simulink model "paper1_cs"  (R2021b)
settings: Solver=ode4  StartTime=0.0  StopTime=120  FixedStep=1/20  RelTol=1e-3
PreLoadFcn:
  | mbxruntime.callbacks.PreLoadFcn(bdroot);
PostLoadFcn:
  | mbxruntime.callbacks.PostLoadFcn(bdroot);
InitFcn:
  | mbxruntime.callbacks.InitFcn(bdroot);
StartFcn:
  | mbxruntime.callbacks.StartFcn(bdroot);
StopFcn:
  | mbxruntime.callbacks.StopFcn(bdroot);
model workspace (MAT data in the model file):
  mbox_table : object (value not decoded)
  model_closed = 0
  sim_status = 0
undefined symbols (not defined in the file): DiscIntNeverNeededParam
libraries: PreScanSimulinkLibrary x12, Solver_SF x6, simulink x1
(part 3 of 3)

== system paper1_cs/Audi_A8_Sedan_5/SELF_Demux ==
  SELF : Inport  OutDataTypeStr=Bus: PRESCAN_SELFSENSORDATA
  Bus Selector : BusSelector  OutputSignals=PositionX,PositionY,PositionZ,OrientationRoll,OrientationPitch,OrientationYaw,Velocity,Yaw_rate,Lat,Long,Alt
  Demux2 : Demux  Outputs=3
  Gain : Gain  Gain=180/pi
  Gain1 : Gain  Gain=180/pi
  Vector Concatenate1 : Concatenate  NumInputs=3
  compas converter : Subsystem
  x [m] : Outport
  y [m] : Outport  Port=2
  z [m] : Outport  Port=3
  rotx [deg] : Outport  Port=4
  roty [deg] : Outport  Port=5
  rotz [deg] : Outport  Port=6
  GPS lat [deg] : Outport  Port=7
  GPS long [deg] : Outport  Port=8
  GPS alt [m] : Outport  Port=9
  velocity [m/s] : Outport  Port=10
  heading [deg] : Outport  Port=11
  yaw rate [deg/s] : Outport  Port=12
  wires:
  Bus Selector/11 -> GPS alt [m]/1  "<Alt>"
  Bus Selector/10 -> GPS long [deg]/1  "<Long>"
  Bus Selector/9 -> GPS lat [deg]/1  "<Lat>"
  Bus Selector/8 -> Gain1/1  "<Yaw_rate>"
  Bus Selector/7 -> velocity [m/s]/1  "<Velocity>"
  Bus Selector/6 -> compas converter/1(rotz [rad]), Vector Concatenate1/3  "<OrientationYaw>"
  Bus Selector/5 -> Vector Concatenate1/2  "<OrientationPitch>"
  Bus Selector/4 -> Vector Concatenate1/1  "<OrientationRoll>"
  Vector Concatenate1/1 -> Gain/1
  Bus Selector/3 -> z [m]/1  "<PositionZ>"
  Bus Selector/2 -> y [m]/1  "<PositionY>"
  Bus Selector/1 -> x [m]/1  "<PositionX>"
  SELF/1 -> Bus Selector/1
  Gain/1 -> Demux2/1
  Demux2/1 -> rotx [deg]/1
  Demux2/2 -> roty [deg]/1
  Demux2/3 -> rotz [deg]/1
  compas converter/1(heading [deg]) -> heading [deg]/1
  Gain1/1 -> yaw rate [deg/s]/1

== system paper1_cs/Audi_A8_Sedan_5/STATE_Audi_A8_Sedan_5 ==
  State : Inport  SampleTime=TimeStep
  Bus Creator : BusCreator  Inputs=15  OutDataTypeStr=Bus: PRESCAN_STATEACTUATORDATA  NonVirtualBus=on
  Demux : Demux  Outputs=15
  iniBODYAngles wrtVEH [rad] : Constant  Value=[Roll0 Pitch0 0]  SampleTime=TimeStep
  iniVEHAngles wrtGLOB [rad] : Constant  Value=[0 0 Yaw0]  SampleTime=TimeStep
  iniVEHposition wrtGLOB [m] : Constant  Value=[x0 y0 z0]  SampleTime=TimeStep
  state2FullState : PreScanSimulinkLibrary/state2FullState  SystemSampleTime=-1  VariantActivationTime=update diagram  Latency=0  AutoFrameSizeCalculation=off
  StateBus : Outport  OutDataTypeStr=Bus: PRESCAN_STATEACTUATORDATA
  wires:
  Bus Creator/1 -> StateBus/1
  State/1 -> state2FullState/1
  state2FullState/1 -> Demux/1
  iniVEHposition wrtGLOB [m]/1 -> state2FullState/2
  iniBODYAngles wrtVEH [rad]/1 -> state2FullState/3
  iniVEHAngles wrtGLOB [rad]/1 -> state2FullState/4
  Demux/1 -> Bus Creator/1  "PositionX"
  Demux/2 -> Bus Creator/2  "PositionY"
  Demux/3 -> Bus Creator/3  "PositionZ"
  Demux/4 -> Bus Creator/4  "VelocityX"
  Demux/5 -> Bus Creator/5  "VelocityY"
  Demux/6 -> Bus Creator/6  "VelocityZ"
  Demux/7 -> Bus Creator/7  "AccelerationX"
  Demux/8 -> Bus Creator/8  "AccelerationY"
  Demux/9 -> Bus Creator/9  "AccelerationZ"
  Demux/10 -> Bus Creator/10  "OrientationRoll"
  Demux/11 -> Bus Creator/11  "OrientationPitch"
  Demux/12 -> Bus Creator/12  "OrientationYaw"
  Demux/13 -> Bus Creator/13  "AngularVelocityRoll"
  Demux/14 -> Bus Creator/14  "AngularVelocityPitch"
  Demux/15 -> Bus Creator/15  "AngularVelocityYaw"

== system paper1_cs/Audi_A8_Sedan_6/Dynamics_UserSpecified ==
  note: For state mode 'Dynamic' positions
      | are not taken into account, as they
      | are computed by integrating velocity.
      | Click annotation for Help.
  CarSim S-Function : Solver_SF/CarSim S-Function  Priority=1  Commented=on  SIMFILE=simfile.sim  Run_RTs=off  vs_state_ind=Run  StopMode_ind=Vehicle Model
  Ground1 : Ground
  MuxState : Subsystem  Tag=mux/State  mask(Empty Dynamics State Block){positioningmode=on, TimeStep=1/20}
      mask prompts: positioningmode "Positioning Mode"; TimeStep "Auto Assigned: Time Step [s]"
      mask help:
      | Build the state of an actor based on user input.
      | The user can either use positioning mode or dynamics mode.
      | - When using positioning mode the position and orientation of the actor are set directly based on the input. Expected input is relative to the initial position and orientation of the actor. It's also possible to specify the velocity of the actor, though this input isn't used, only passed on.
      | - When using dynamics mode the position input is ignored. Expected input is velocity and orientation. The velocity is relative the current orientation of the actor, while orientation is relative to its initial orientation. The position of the actor is calculated based on the velocity and orientation given.
      settings: DeleteFcn=PreScanBlockDeleteFcn;
  State : Outport
  wires:
  [v6] -> MuxState/4(dx [m/s])
  [x6] -> MuxState/1(x [m])
  MuxState/1(state) -> State/1
  Ground1/1 -> MuxState/2(y [m]), MuxState/3(z [m]), MuxState/5(dy [m/s]), MuxState/6(dz [m/s]), MuxState/7(R [rad]), MuxState/8(P [rad]), MuxState/9(Y [rad])

== system paper1_cs/Audi_A8_Sedan_6/SELF_Demux ==
  SELF : Inport  OutDataTypeStr=Bus: PRESCAN_SELFSENSORDATA
  Bus Selector : BusSelector  OutputSignals=PositionX,PositionY,PositionZ,OrientationRoll,OrientationPitch,OrientationYaw,Velocity,Yaw_rate,Lat,Long,Alt
  Demux2 : Demux  Outputs=3
  Gain : Gain  Gain=180/pi
  Gain1 : Gain  Gain=180/pi
  Vector Concatenate1 : Concatenate  NumInputs=3
  compas converter : Subsystem
  x [m] : Outport
  y [m] : Outport  Port=2
  z [m] : Outport  Port=3
  rotx [deg] : Outport  Port=4
  roty [deg] : Outport  Port=5
  rotz [deg] : Outport  Port=6
  GPS lat [deg] : Outport  Port=7
  GPS long [deg] : Outport  Port=8
  GPS alt [m] : Outport  Port=9
  velocity [m/s] : Outport  Port=10
  heading [deg] : Outport  Port=11
  yaw rate [deg/s] : Outport  Port=12
  wires:
  Bus Selector/11 -> GPS alt [m]/1  "<Alt>"
  Bus Selector/10 -> GPS long [deg]/1  "<Long>"
  Bus Selector/9 -> GPS lat [deg]/1  "<Lat>"
  Bus Selector/8 -> Gain1/1  "<Yaw_rate>"
  Bus Selector/7 -> velocity [m/s]/1  "<Velocity>"
  Bus Selector/6 -> compas converter/1(rotz [rad]), Vector Concatenate1/3  "<OrientationYaw>"
  Bus Selector/5 -> Vector Concatenate1/2  "<OrientationPitch>"
  Bus Selector/4 -> Vector Concatenate1/1  "<OrientationRoll>"
  Vector Concatenate1/1 -> Gain/1
  Bus Selector/3 -> z [m]/1  "<PositionZ>"
  Bus Selector/2 -> y [m]/1  "<PositionY>"
  Bus Selector/1 -> x [m]/1  "<PositionX>"
  SELF/1 -> Bus Selector/1
  Gain/1 -> Demux2/1
  Demux2/1 -> rotx [deg]/1
  Demux2/2 -> roty [deg]/1
  Demux2/3 -> rotz [deg]/1
  compas converter/1(heading [deg]) -> heading [deg]/1
  Gain1/1 -> yaw rate [deg/s]/1

== system paper1_cs/Audi_A8_Sedan_6/STATE_Audi_A8_Sedan_6 ==
  State : Inport  SampleTime=TimeStep
  Bus Creator : BusCreator  Inputs=15  OutDataTypeStr=Bus: PRESCAN_STATEACTUATORDATA  NonVirtualBus=on
  Demux : Demux  Outputs=15
  iniBODYAngles wrtVEH [rad] : Constant  Value=[Roll0 Pitch0 0]  SampleTime=TimeStep
  iniVEHAngles wrtGLOB [rad] : Constant  Value=[0 0 Yaw0]  SampleTime=TimeStep
  iniVEHposition wrtGLOB [m] : Constant  Value=[x0 y0 z0]  SampleTime=TimeStep
  state2FullState : PreScanSimulinkLibrary/state2FullState  SystemSampleTime=-1  VariantActivationTime=update diagram  Latency=0  AutoFrameSizeCalculation=off
  StateBus : Outport  OutDataTypeStr=Bus: PRESCAN_STATEACTUATORDATA
  wires:
  Bus Creator/1 -> StateBus/1
  State/1 -> state2FullState/1
  state2FullState/1 -> Demux/1
  iniVEHposition wrtGLOB [m]/1 -> state2FullState/2
  iniBODYAngles wrtVEH [rad]/1 -> state2FullState/3
  iniVEHAngles wrtGLOB [rad]/1 -> state2FullState/4
  Demux/1 -> Bus Creator/1  "PositionX"
  Demux/2 -> Bus Creator/2  "PositionY"
  Demux/3 -> Bus Creator/3  "PositionZ"
  Demux/4 -> Bus Creator/4  "VelocityX"
  Demux/5 -> Bus Creator/5  "VelocityY"
  Demux/6 -> Bus Creator/6  "VelocityZ"
  Demux/7 -> Bus Creator/7  "AccelerationX"
  Demux/8 -> Bus Creator/8  "AccelerationY"
  Demux/9 -> Bus Creator/9  "AccelerationZ"
  Demux/10 -> Bus Creator/10  "OrientationRoll"
  Demux/11 -> Bus Creator/11  "OrientationPitch"
  Demux/12 -> Bus Creator/12  "OrientationYaw"
  Demux/13 -> Bus Creator/13  "AngularVelocityRoll"
  Demux/14 -> Bus Creator/14  "AngularVelocityPitch"
  Demux/15 -> Bus Creator/15  "AngularVelocityYaw"

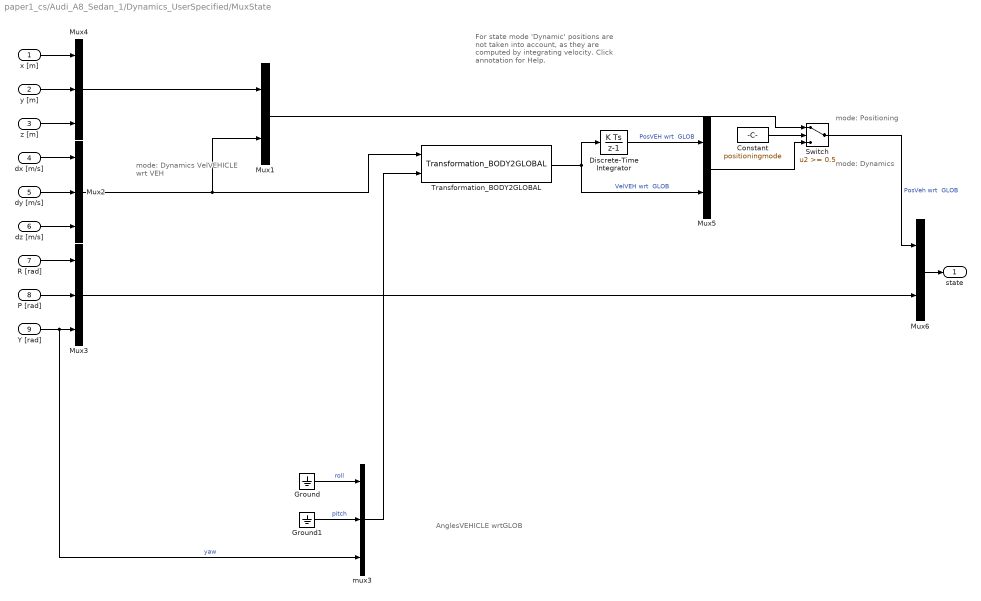
== system paper1_cs/Audi_A8_Sedan_1/Dynamics_UserSpecified/MuxState ==
  note: mode: Dynamics
  note: mode: Positioning
  note: mode: Dynamics
      | VelVEHICLE
      | wrt VEH
  note: AnglesVEHICLE
      | wrtGLOB
  note: For state mode 'Dynamic' positions
      | are not taken into account, as they
      | are computed by integrating velocity.
      | Click annotation for Help.
  x [m] : Inport  SampleTime=TimeStep
  y [m] : Inport  Port=2  SampleTime=TimeStep
  z [m] : Inport  Port=3  SampleTime=TimeStep
  dx [m/s] : Inport  Port=4  SampleTime=TimeStep
  dy [m/s] : Inport  Port=5  SampleTime=TimeStep
  dz [m/s] : Inport  Port=6  SampleTime=TimeStep
  R [rad] : Inport  Port=7  SampleTime=TimeStep
  P [rad] : Inport  Port=8  SampleTime=TimeStep
  Y [rad] : Inport  Port=9  SampleTime=TimeStep
  Constant : Constant  DisableCoverage=on  Value=positioningmode
  Discrete-Time Integrator : DiscreteIntegrator  SampleTime=TimeStep  ICPrevOutput=DiscIntNeverNeededParam  ICPrevScaledInput=DiscIntNeverNeededParam
  Ground : Ground
  Ground1 : Ground
  Mux1 : Mux  Inputs=[3 3]
  Mux2 : Mux  Inputs=3
  Mux3 : Mux  Inputs=3
  Mux4 : Mux  Inputs=3
  Mux5 : Mux  Inputs=[3 3]
  Mux6 : Mux  Inputs=[6 3]
  Switch : Switch  Threshold=0.5
  Transformation_BODY2GLOBAL : PreScanSimulinkLibrary/Simple_Vehicle_Dynamics/Chassis/MuxDynState/Transformation_BODY2GLOBAL  SystemSampleTime=-1  VariantActivationTime=update diagram  Latency=0  AutoFrameSizeCalculation=off
  mux3 : Mux  Inputs=3
  state : Outport
  wires:
  Constant/1 -> Switch/2
  Mux6/1 -> state/1
  Mux4/1 -> Mux1/1
  Mux5/1 -> Switch/3
  Mux1/1 -> Switch/1
  Switch/1 -> Mux6/1  "PosVeh wrt  GLOB"
  P [rad]/1 -> Mux3/2
  R [rad]/1 -> Mux3/1
  dz [m/s]/1 -> Mux2/3
  dy [m/s]/1 -> Mux2/2
  dx [m/s]/1 -> Mux2/1
  z [m]/1 -> Mux4/3
  y [m]/1 -> Mux4/2
  x [m]/1 -> Mux4/1
  Ground1/1 -> mux3/2  "pitch"
  Y [rad]/1 -> mux3/3, Mux3/3  "yaw"
  Mux3/1 -> Mux6/2
  Transformation_BODY2GLOBAL/1 -> Discrete-Time Integrator/1, Mux5/2  "VelVEH wrt  GLOB"
  mux3/1 -> Transformation_BODY2GLOBAL/2
  Ground/1 -> mux3/1  "roll"
  Mux2/1 -> Mux1/2, Transformation_BODY2GLOBAL/1
  Discrete-Time Integrator/1 -> Mux5/1  "PosVEH wrt  GLOB"

== system paper1_cs/Audi_A8_Sedan_1/SELF_Demux/compas converter ==
  rotz [rad] : Inport
  cart2compas : Subsystem
  rad2deg : Gain  Gain=180/pi
  heading [deg] : Outport
  wires:
  rad2deg/1 -> cart2compas/1(Angle [deg])
  rotz [rad]/1 -> rad2deg/1
  cart2compas/1(heading [deg]) -> heading [deg]/1

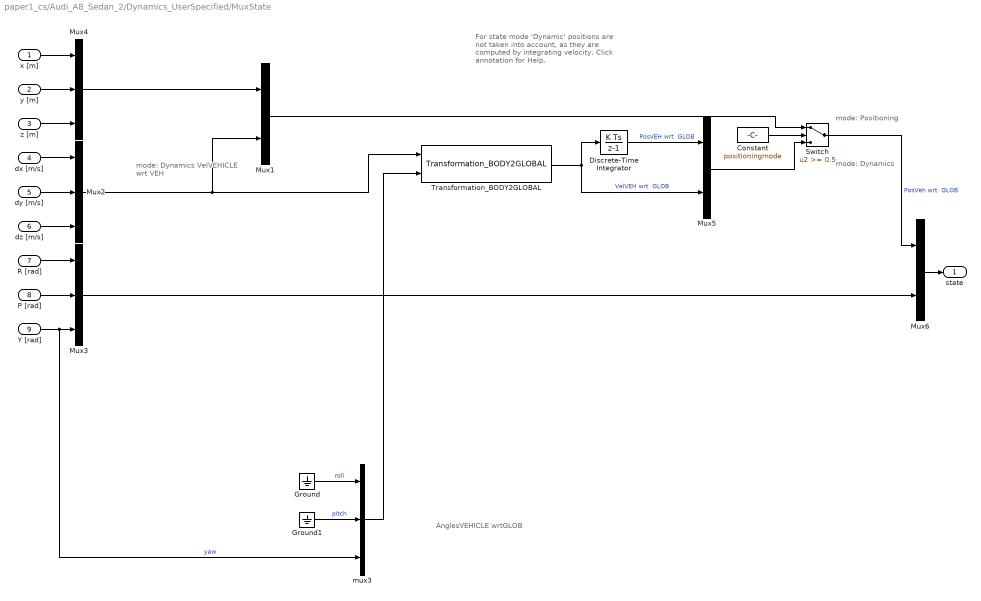
== system paper1_cs/Audi_A8_Sedan_2/Dynamics_UserSpecified/MuxState ==
  note: mode: Dynamics
  note: mode: Positioning
  note: mode: Dynamics
      | VelVEHICLE
      | wrt VEH
  note: AnglesVEHICLE
      | wrtGLOB
  note: For state mode 'Dynamic' positions
      | are not taken into account, as they
      | are computed by integrating velocity.
      | Click annotation for Help.
  x [m] : Inport  SampleTime=TimeStep
  y [m] : Inport  Port=2  SampleTime=TimeStep
  z [m] : Inport  Port=3  SampleTime=TimeStep
  dx [m/s] : Inport  Port=4  SampleTime=TimeStep
  dy [m/s] : Inport  Port=5  SampleTime=TimeStep
  dz [m/s] : Inport  Port=6  SampleTime=TimeStep
  R [rad] : Inport  Port=7  SampleTime=TimeStep
  P [rad] : Inport  Port=8  SampleTime=TimeStep
  Y [rad] : Inport  Port=9  SampleTime=TimeStep
  Constant : Constant  DisableCoverage=on  Value=positioningmode
  Discrete-Time Integrator : DiscreteIntegrator  SampleTime=TimeStep  ICPrevOutput=DiscIntNeverNeededParam  ICPrevScaledInput=DiscIntNeverNeededParam
  Ground : Ground
  Ground1 : Ground
  Mux1 : Mux  Inputs=[3 3]
  Mux2 : Mux  Inputs=3
  Mux3 : Mux  Inputs=3
  Mux4 : Mux  Inputs=3
  Mux5 : Mux  Inputs=[3 3]
  Mux6 : Mux  Inputs=[6 3]
  Switch : Switch  Threshold=0.5
  Transformation_BODY2GLOBAL : PreScanSimulinkLibrary/Simple_Vehicle_Dynamics/Chassis/MuxDynState/Transformation_BODY2GLOBAL  SystemSampleTime=-1  VariantActivationTime=update diagram  Latency=0  AutoFrameSizeCalculation=off
  mux3 : Mux  Inputs=3
  state : Outport
  wires:
  Constant/1 -> Switch/2
  Mux6/1 -> state/1
  Mux4/1 -> Mux1/1
  Mux5/1 -> Switch/3
  Mux1/1 -> Switch/1
  Switch/1 -> Mux6/1  "PosVeh wrt  GLOB"
  P [rad]/1 -> Mux3/2
  R [rad]/1 -> Mux3/1
  dz [m/s]/1 -> Mux2/3
  dy [m/s]/1 -> Mux2/2
  dx [m/s]/1 -> Mux2/1
  z [m]/1 -> Mux4/3
  y [m]/1 -> Mux4/2
  x [m]/1 -> Mux4/1
  Ground1/1 -> mux3/2  "pitch"
  Y [rad]/1 -> mux3/3, Mux3/3  "yaw"
  Mux3/1 -> Mux6/2
  Transformation_BODY2GLOBAL/1 -> Discrete-Time Integrator/1, Mux5/2  "VelVEH wrt  GLOB"
  mux3/1 -> Transformation_BODY2GLOBAL/2
  Ground/1 -> mux3/1  "roll"
  Mux2/1 -> Mux1/2, Transformation_BODY2GLOBAL/1
  Discrete-Time Integrator/1 -> Mux5/1  "PosVEH wrt  GLOB"

== system paper1_cs/Audi_A8_Sedan_2/SELF_Demux/compas converter ==
  rotz [rad] : Inport
  cart2compas : Subsystem
  rad2deg : Gain  Gain=180/pi
  heading [deg] : Outport
  wires:
  rad2deg/1 -> cart2compas/1(Angle [deg])
  rotz [rad]/1 -> rad2deg/1
  cart2compas/1(heading [deg]) -> heading [deg]/1

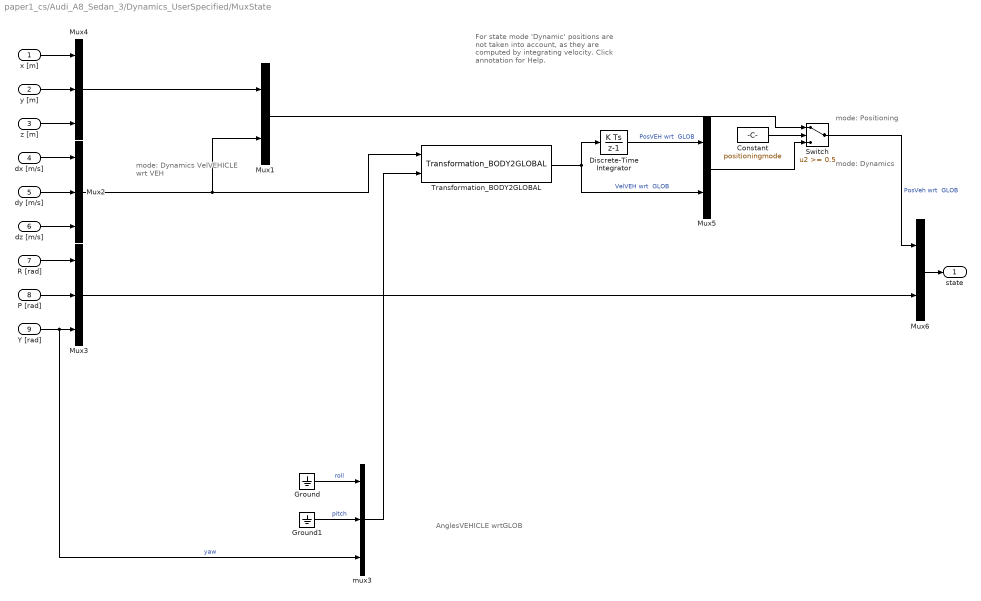
== system paper1_cs/Audi_A8_Sedan_3/Dynamics_UserSpecified/MuxState ==
  note: mode: Dynamics
  note: mode: Positioning
  note: mode: Dynamics
      | VelVEHICLE
      | wrt VEH
  note: AnglesVEHICLE
      | wrtGLOB
  note: For state mode 'Dynamic' positions
      | are not taken into account, as they
      | are computed by integrating velocity.
      | Click annotation for Help.
  x [m] : Inport  SampleTime=TimeStep
  y [m] : Inport  Port=2  SampleTime=TimeStep
  z [m] : Inport  Port=3  SampleTime=TimeStep
  dx [m/s] : Inport  Port=4  SampleTime=TimeStep
  dy [m/s] : Inport  Port=5  SampleTime=TimeStep
  dz [m/s] : Inport  Port=6  SampleTime=TimeStep
  R [rad] : Inport  Port=7  SampleTime=TimeStep
  P [rad] : Inport  Port=8  SampleTime=TimeStep
  Y [rad] : Inport  Port=9  SampleTime=TimeStep
  Constant : Constant  DisableCoverage=on  Value=positioningmode
  Discrete-Time Integrator : DiscreteIntegrator  SampleTime=TimeStep  ICPrevOutput=DiscIntNeverNeededParam  ICPrevScaledInput=DiscIntNeverNeededParam
  Ground : Ground
  Ground1 : Ground
  Mux1 : Mux  Inputs=[3 3]
  Mux2 : Mux  Inputs=3
  Mux3 : Mux  Inputs=3
  Mux4 : Mux  Inputs=3
  Mux5 : Mux  Inputs=[3 3]
  Mux6 : Mux  Inputs=[6 3]
  Switch : Switch  Threshold=0.5
  Transformation_BODY2GLOBAL : PreScanSimulinkLibrary/Simple_Vehicle_Dynamics/Chassis/MuxDynState/Transformation_BODY2GLOBAL  SystemSampleTime=-1  VariantActivationTime=update diagram  Latency=0  AutoFrameSizeCalculation=off
  mux3 : Mux  Inputs=3
  state : Outport
  wires:
  Constant/1 -> Switch/2
  Mux6/1 -> state/1
  Mux4/1 -> Mux1/1
  Mux5/1 -> Switch/3
  Mux1/1 -> Switch/1
  Switch/1 -> Mux6/1  "PosVeh wrt  GLOB"
  P [rad]/1 -> Mux3/2
  R [rad]/1 -> Mux3/1
  dz [m/s]/1 -> Mux2/3
  dy [m/s]/1 -> Mux2/2
  dx [m/s]/1 -> Mux2/1
  z [m]/1 -> Mux4/3
  y [m]/1 -> Mux4/2
  x [m]/1 -> Mux4/1
  Ground1/1 -> mux3/2  "pitch"
  Y [rad]/1 -> mux3/3, Mux3/3  "yaw"
  Mux3/1 -> Mux6/2
  Transformation_BODY2GLOBAL/1 -> Discrete-Time Integrator/1, Mux5/2  "VelVEH wrt  GLOB"
  mux3/1 -> Transformation_BODY2GLOBAL/2
  Ground/1 -> mux3/1  "roll"
  Mux2/1 -> Mux1/2, Transformation_BODY2GLOBAL/1
  Discrete-Time Integrator/1 -> Mux5/1  "PosVEH wrt  GLOB"

== system paper1_cs/Audi_A8_Sedan_3/SELF_Demux/compas converter ==
  rotz [rad] : Inport
  cart2compas : Subsystem
  rad2deg : Gain  Gain=180/pi
  heading [deg] : Outport
  wires:
  rad2deg/1 -> cart2compas/1(Angle [deg])
  rotz [rad]/1 -> rad2deg/1
  cart2compas/1(heading [deg]) -> heading [deg]/1

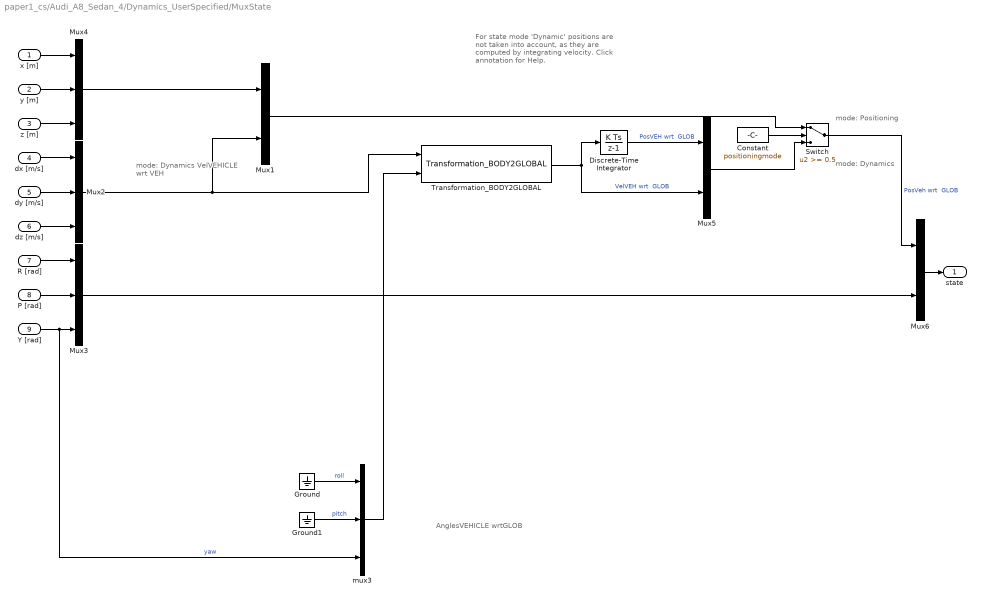
== system paper1_cs/Audi_A8_Sedan_4/Dynamics_UserSpecified/MuxState ==
  note: mode: Dynamics
  note: mode: Positioning
  note: mode: Dynamics
      | VelVEHICLE
      | wrt VEH
  note: AnglesVEHICLE
      | wrtGLOB
  note: For state mode 'Dynamic' positions
      | are not taken into account, as they
      | are computed by integrating velocity.
      | Click annotation for Help.
  x [m] : Inport  SampleTime=TimeStep
  y [m] : Inport  Port=2  SampleTime=TimeStep
  z [m] : Inport  Port=3  SampleTime=TimeStep
  dx [m/s] : Inport  Port=4  SampleTime=TimeStep
  dy [m/s] : Inport  Port=5  SampleTime=TimeStep
  dz [m/s] : Inport  Port=6  SampleTime=TimeStep
  R [rad] : Inport  Port=7  SampleTime=TimeStep
  P [rad] : Inport  Port=8  SampleTime=TimeStep
  Y [rad] : Inport  Port=9  SampleTime=TimeStep
  Constant : Constant  DisableCoverage=on  Value=positioningmode
  Discrete-Time Integrator : DiscreteIntegrator  SampleTime=TimeStep  ICPrevOutput=DiscIntNeverNeededParam  ICPrevScaledInput=DiscIntNeverNeededParam
  Ground : Ground
  Ground1 : Ground
  Mux1 : Mux  Inputs=[3 3]
  Mux2 : Mux  Inputs=3
  Mux3 : Mux  Inputs=3
  Mux4 : Mux  Inputs=3
  Mux5 : Mux  Inputs=[3 3]
  Mux6 : Mux  Inputs=[6 3]
  Switch : Switch  Threshold=0.5
  Transformation_BODY2GLOBAL : PreScanSimulinkLibrary/Simple_Vehicle_Dynamics/Chassis/MuxDynState/Transformation_BODY2GLOBAL  SystemSampleTime=-1  VariantActivationTime=update diagram  Latency=0  AutoFrameSizeCalculation=off
  mux3 : Mux  Inputs=3
  state : Outport
  wires:
  Constant/1 -> Switch/2
  Mux6/1 -> state/1
  Mux4/1 -> Mux1/1
  Mux5/1 -> Switch/3
  Mux1/1 -> Switch/1
  Switch/1 -> Mux6/1  "PosVeh wrt  GLOB"
  P [rad]/1 -> Mux3/2
  R [rad]/1 -> Mux3/1
  dz [m/s]/1 -> Mux2/3
  dy [m/s]/1 -> Mux2/2
  dx [m/s]/1 -> Mux2/1
  z [m]/1 -> Mux4/3
  y [m]/1 -> Mux4/2
  x [m]/1 -> Mux4/1
  Ground1/1 -> mux3/2  "pitch"
  Y [rad]/1 -> mux3/3, Mux3/3  "yaw"
  Mux3/1 -> Mux6/2
  Transformation_BODY2GLOBAL/1 -> Discrete-Time Integrator/1, Mux5/2  "VelVEH wrt  GLOB"
  mux3/1 -> Transformation_BODY2GLOBAL/2
  Ground/1 -> mux3/1  "roll"
  Mux2/1 -> Mux1/2, Transformation_BODY2GLOBAL/1
  Discrete-Time Integrator/1 -> Mux5/1  "PosVEH wrt  GLOB"

== system paper1_cs/Audi_A8_Sedan_4/SELF_Demux/compas converter ==
  rotz [rad] : Inport
  cart2compas : Subsystem
  rad2deg : Gain  Gain=180/pi
  heading [deg] : Outport
  wires:
  rad2deg/1 -> cart2compas/1(Angle [deg])
  rotz [rad]/1 -> rad2deg/1
  cart2compas/1(heading [deg]) -> heading [deg]/1

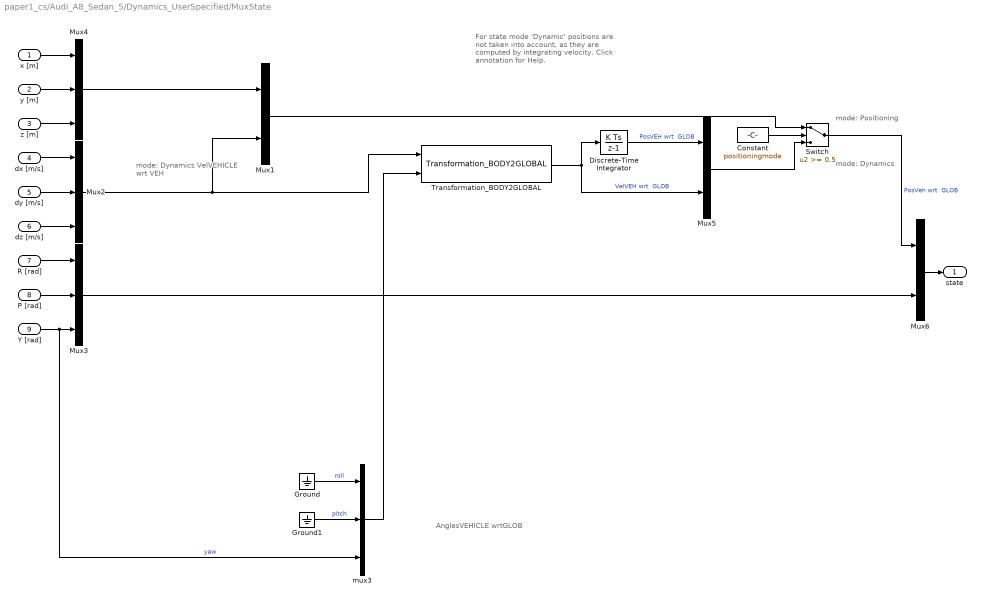
== system paper1_cs/Audi_A8_Sedan_5/Dynamics_UserSpecified/MuxState ==
  note: mode: Dynamics
  note: mode: Positioning
  note: mode: Dynamics
      | VelVEHICLE
      | wrt VEH
  note: AnglesVEHICLE
      | wrtGLOB
  note: For state mode 'Dynamic' positions
      | are not taken into account, as they
      | are computed by integrating velocity.
      | Click annotation for Help.
  x [m] : Inport  SampleTime=TimeStep
  y [m] : Inport  Port=2  SampleTime=TimeStep
  z [m] : Inport  Port=3  SampleTime=TimeStep
  dx [m/s] : Inport  Port=4  SampleTime=TimeStep
  dy [m/s] : Inport  Port=5  SampleTime=TimeStep
  dz [m/s] : Inport  Port=6  SampleTime=TimeStep
  R [rad] : Inport  Port=7  SampleTime=TimeStep
  P [rad] : Inport  Port=8  SampleTime=TimeStep
  Y [rad] : Inport  Port=9  SampleTime=TimeStep
  Constant : Constant  DisableCoverage=on  Value=positioningmode
  Discrete-Time Integrator : DiscreteIntegrator  SampleTime=TimeStep  ICPrevOutput=DiscIntNeverNeededParam  ICPrevScaledInput=DiscIntNeverNeededParam
  Ground : Ground
  Ground1 : Ground
  Mux1 : Mux  Inputs=[3 3]
  Mux2 : Mux  Inputs=3
  Mux3 : Mux  Inputs=3
  Mux4 : Mux  Inputs=3
  Mux5 : Mux  Inputs=[3 3]
  Mux6 : Mux  Inputs=[6 3]
  Switch : Switch  Threshold=0.5
  Transformation_BODY2GLOBAL : PreScanSimulinkLibrary/Simple_Vehicle_Dynamics/Chassis/MuxDynState/Transformation_BODY2GLOBAL  SystemSampleTime=-1  VariantActivationTime=update diagram  Latency=0  AutoFrameSizeCalculation=off
  mux3 : Mux  Inputs=3
  state : Outport
  wires:
  Constant/1 -> Switch/2
  Mux6/1 -> state/1
  Mux4/1 -> Mux1/1
  Mux5/1 -> Switch/3
  Mux1/1 -> Switch/1
  Switch/1 -> Mux6/1  "PosVeh wrt  GLOB"
  P [rad]/1 -> Mux3/2
  R [rad]/1 -> Mux3/1
  dz [m/s]/1 -> Mux2/3
  dy [m/s]/1 -> Mux2/2
  dx [m/s]/1 -> Mux2/1
  z [m]/1 -> Mux4/3
  y [m]/1 -> Mux4/2
  x [m]/1 -> Mux4/1
  Ground1/1 -> mux3/2  "pitch"
  Y [rad]/1 -> mux3/3, Mux3/3  "yaw"
  Mux3/1 -> Mux6/2
  Transformation_BODY2GLOBAL/1 -> Discrete-Time Integrator/1, Mux5/2  "VelVEH wrt  GLOB"
  mux3/1 -> Transformation_BODY2GLOBAL/2
  Ground/1 -> mux3/1  "roll"
  Mux2/1 -> Mux1/2, Transformation_BODY2GLOBAL/1
  Discrete-Time Integrator/1 -> Mux5/1  "PosVEH wrt  GLOB"

== system paper1_cs/Audi_A8_Sedan_5/SELF_Demux/compas converter ==
  rotz [rad] : Inport
  cart2compas : Subsystem
  rad2deg : Gain  Gain=180/pi
  heading [deg] : Outport
  wires:
  rad2deg/1 -> cart2compas/1(Angle [deg])
  rotz [rad]/1 -> rad2deg/1
  cart2compas/1(heading [deg]) -> heading [deg]/1

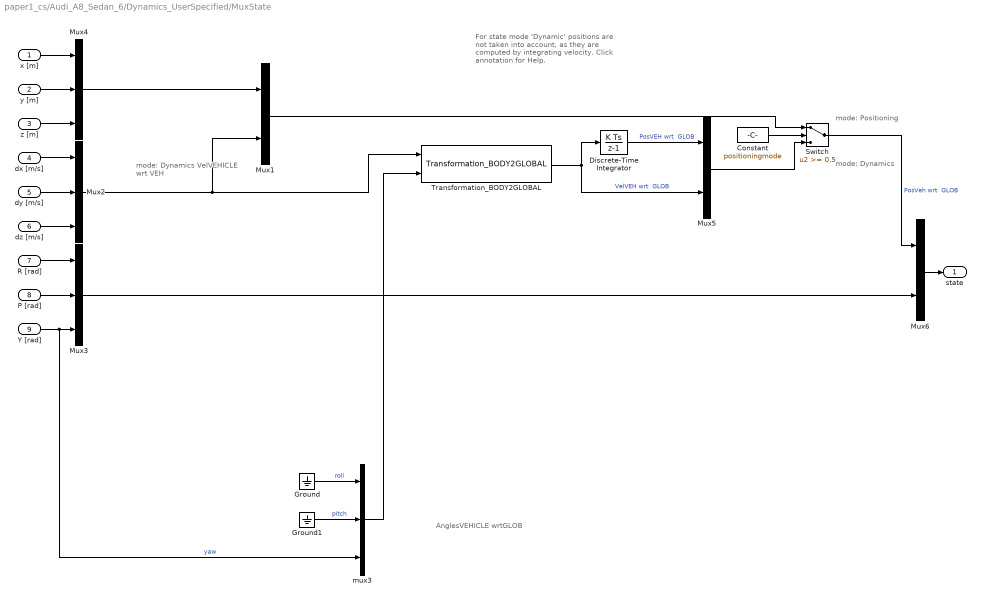
== system paper1_cs/Audi_A8_Sedan_6/Dynamics_UserSpecified/MuxState ==
  note: mode: Dynamics
  note: mode: Positioning
  note: mode: Dynamics
      | VelVEHICLE
      | wrt VEH
  note: AnglesVEHICLE
      | wrtGLOB
  note: For state mode 'Dynamic' positions
      | are not taken into account, as they
      | are computed by integrating velocity.
      | Click annotation for Help.
  x [m] : Inport  SampleTime=TimeStep
  y [m] : Inport  Port=2  SampleTime=TimeStep
  z [m] : Inport  Port=3  SampleTime=TimeStep
  dx [m/s] : Inport  Port=4  SampleTime=TimeStep
  dy [m/s] : Inport  Port=5  SampleTime=TimeStep
  dz [m/s] : Inport  Port=6  SampleTime=TimeStep
  R [rad] : Inport  Port=7  SampleTime=TimeStep
  P [rad] : Inport  Port=8  SampleTime=TimeStep
  Y [rad] : Inport  Port=9  SampleTime=TimeStep
  Constant : Constant  DisableCoverage=on  Value=positioningmode
  Discrete-Time Integrator : DiscreteIntegrator  SampleTime=TimeStep  ICPrevOutput=DiscIntNeverNeededParam  ICPrevScaledInput=DiscIntNeverNeededParam
  Ground : Ground
  Ground1 : Ground
  Mux1 : Mux  Inputs=[3 3]
  Mux2 : Mux  Inputs=3
  Mux3 : Mux  Inputs=3
  Mux4 : Mux  Inputs=3
  Mux5 : Mux  Inputs=[3 3]
  Mux6 : Mux  Inputs=[6 3]
  Switch : Switch  Threshold=0.5
  Transformation_BODY2GLOBAL : PreScanSimulinkLibrary/Simple_Vehicle_Dynamics/Chassis/MuxDynState/Transformation_BODY2GLOBAL  SystemSampleTime=-1  VariantActivationTime=update diagram  Latency=0  AutoFrameSizeCalculation=off
  mux3 : Mux  Inputs=3
  state : Outport
  wires:
  Constant/1 -> Switch/2
  Mux6/1 -> state/1
  Mux4/1 -> Mux1/1
  Mux5/1 -> Switch/3
  Mux1/1 -> Switch/1
  Switch/1 -> Mux6/1  "PosVeh wrt  GLOB"
  P [rad]/1 -> Mux3/2
  R [rad]/1 -> Mux3/1
  dz [m/s]/1 -> Mux2/3
  dy [m/s]/1 -> Mux2/2
  dx [m/s]/1 -> Mux2/1
  z [m]/1 -> Mux4/3
  y [m]/1 -> Mux4/2
  x [m]/1 -> Mux4/1
  Ground1/1 -> mux3/2  "pitch"
  Y [rad]/1 -> mux3/3, Mux3/3  "yaw"
  Mux3/1 -> Mux6/2
  Transformation_BODY2GLOBAL/1 -> Discrete-Time Integrator/1, Mux5/2  "VelVEH wrt  GLOB"
  mux3/1 -> Transformation_BODY2GLOBAL/2
  Ground/1 -> mux3/1  "roll"
  Mux2/1 -> Mux1/2, Transformation_BODY2GLOBAL/1
  Discrete-Time Integrator/1 -> Mux5/1  "PosVEH wrt  GLOB"

== system paper1_cs/Audi_A8_Sedan_6/SELF_Demux/compas converter ==
  rotz [rad] : Inport
  cart2compas : Subsystem
  rad2deg : Gain  Gain=180/pi
  heading [deg] : Outport
  wires:
  rad2deg/1 -> cart2compas/1(Angle [deg])
  rotz [rad]/1 -> rad2deg/1
  cart2compas/1(heading [deg]) -> heading [deg]/1

== system paper1_cs/Audi_A8_Sedan_1/SELF_Demux/compas converter/cart2compas ==
  Angle [deg] : Inport
  Constant : Constant  Value=90
  Constant1 : Constant  Value=360
  Gain : Gain  Gain=1/360
  Gain1 : Gain  Gain=360
  Gain2 : Gain  Gain=-1
  Rounding Function : Rounding
  Sum : Sum  Inputs=|-+
  Sum1 : Sum  Inputs=-+|
  Sum2 : Sum  Inputs=++|
  heading [deg] : Outport
  wires:
  Gain/1 -> Rounding Function/1
  Rounding Function/1 -> Gain1/1
  Gain1/1 -> Sum/1
  Angle [deg]/1 -> Sum1/2
  Sum/1 -> Gain2/1
  Sum1/1 -> Gain/1, Sum/2
  Constant/1 -> Sum1/1
  Gain2/1 -> Sum2/2
  Constant1/1 -> Sum2/1
  Sum2/1 -> heading [deg]/1

== system paper1_cs/Audi_A8_Sedan_2/SELF_Demux/compas converter/cart2compas ==
  Angle [deg] : Inport
  Constant : Constant  Value=90
  Constant1 : Constant  Value=360
  Gain : Gain  Gain=1/360
  Gain1 : Gain  Gain=360
  Gain2 : Gain  Gain=-1
  Rounding Function : Rounding
  Sum : Sum  Inputs=|-+
  Sum1 : Sum  Inputs=-+|
  Sum2 : Sum  Inputs=++|
  heading [deg] : Outport
  wires:
  Gain/1 -> Rounding Function/1
  Rounding Function/1 -> Gain1/1
  Gain1/1 -> Sum/1
  Angle [deg]/1 -> Sum1/2
  Sum/1 -> Gain2/1
  Sum1/1 -> Gain/1, Sum/2
  Constant/1 -> Sum1/1
  Gain2/1 -> Sum2/2
  Constant1/1 -> Sum2/1
  Sum2/1 -> heading [deg]/1

== system paper1_cs/Audi_A8_Sedan_3/SELF_Demux/compas converter/cart2compas ==
  Angle [deg] : Inport
  Constant : Constant  Value=90
  Constant1 : Constant  Value=360
  Gain : Gain  Gain=1/360
  Gain1 : Gain  Gain=360
  Gain2 : Gain  Gain=-1
  Rounding Function : Rounding
  Sum : Sum  Inputs=|-+
  Sum1 : Sum  Inputs=-+|
  Sum2 : Sum  Inputs=++|
  heading [deg] : Outport
  wires:
  Gain/1 -> Rounding Function/1
  Rounding Function/1 -> Gain1/1
  Gain1/1 -> Sum/1
  Angle [deg]/1 -> Sum1/2
  Sum/1 -> Gain2/1
  Sum1/1 -> Gain/1, Sum/2
  Constant/1 -> Sum1/1
  Gain2/1 -> Sum2/2
  Constant1/1 -> Sum2/1
  Sum2/1 -> heading [deg]/1

== system paper1_cs/Audi_A8_Sedan_4/SELF_Demux/compas converter/cart2compas ==
  Angle [deg] : Inport
  Constant : Constant  Value=90
  Constant1 : Constant  Value=360
  Gain : Gain  Gain=1/360
  Gain1 : Gain  Gain=360
  Gain2 : Gain  Gain=-1
  Rounding Function : Rounding
  Sum : Sum  Inputs=|-+
  Sum1 : Sum  Inputs=-+|
  Sum2 : Sum  Inputs=++|
  heading [deg] : Outport
  wires:
  Gain/1 -> Rounding Function/1
  Rounding Function/1 -> Gain1/1
  Gain1/1 -> Sum/1
  Angle [deg]/1 -> Sum1/2
  Sum/1 -> Gain2/1
  Sum1/1 -> Gain/1, Sum/2
  Constant/1 -> Sum1/1
  Gain2/1 -> Sum2/2
  Constant1/1 -> Sum2/1
  Sum2/1 -> heading [deg]/1

== system paper1_cs/Audi_A8_Sedan_5/SELF_Demux/compas converter/cart2compas ==
  Angle [deg] : Inport
  Constant : Constant  Value=90
  Constant1 : Constant  Value=360
  Gain : Gain  Gain=1/360
  Gain1 : Gain  Gain=360
  Gain2 : Gain  Gain=-1
  Rounding Function : Rounding
  Sum : Sum  Inputs=|-+
  Sum1 : Sum  Inputs=-+|
  Sum2 : Sum  Inputs=++|
  heading [deg] : Outport
  wires:
  Gain/1 -> Rounding Function/1
  Rounding Function/1 -> Gain1/1
  Gain1/1 -> Sum/1
  Angle [deg]/1 -> Sum1/2
  Sum/1 -> Gain2/1
  Sum1/1 -> Gain/1, Sum/2
  Constant/1 -> Sum1/1
  Gain2/1 -> Sum2/2
  Constant1/1 -> Sum2/1
  Sum2/1 -> heading [deg]/1

== system paper1_cs/Audi_A8_Sedan_6/SELF_Demux/compas converter/cart2compas ==
  Angle [deg] : Inport
  Constant : Constant  Value=90
  Constant1 : Constant  Value=360
  Gain : Gain  Gain=1/360
  Gain1 : Gain  Gain=360
  Gain2 : Gain  Gain=-1
  Rounding Function : Rounding
  Sum : Sum  Inputs=|-+
  Sum1 : Sum  Inputs=-+|
  Sum2 : Sum  Inputs=++|
  heading [deg] : Outport
  wires:
  Gain/1 -> Rounding Function/1
  Rounding Function/1 -> Gain1/1
  Gain1/1 -> Sum/1
  Angle [deg]/1 -> Sum1/2
  Sum/1 -> Gain2/1
  Sum1/1 -> Gain/1, Sum/2
  Constant/1 -> Sum1/1
  Gain2/1 -> Sum2/2
  Constant1/1 -> Sum2/1
  Sum2/1 -> heading [deg]/1

== matlab function paper1_cs/时序验证模块 ==
  data: t input; y output
function y = fcn(t)
    persistent last_t;
    if isempty(last_t)
        last_t = t;  % 初始化时间
    end
dt = t - last_t;  % 计算时间步长
y= dt;
end

== matlab function paper1_cs/Audi_A8_Sedan_1/MATLAB Function ==
  data: t input; position1 output; v1 output; p input; v input; a input; position0 input; v0 input; position2 input; v2 input
function [position1,v1] = fcn(t,p,v,a,position0,v0,position2,v2)
    % 跟随车1
    % 与虚拟领导者以及后车存在通信
    % 车辆参数          
    m=1.8;                                  %质量
    Tau=0.6;                                %时滞常数
    le=5;                                   %车辆长度
    A=[0 1 0; 0 0 1; 0 0 -1/Tau];           %系统状态矩阵
    ds=15;                                  %期望距离
    dm1=124.9;
    B=[0;0;1/(m*Tau)];                      %控制输入矩阵
    Bn=[0;0;1];
    kd = 0.24;                             %1号车的干扰系数
    car1_ref = [position0-20,v0,0];        %1号车的参考位置
    c = eye(3);
    x1 = [p;v;a];                          %1号车的真实状态
    y1 = c*x1;                             %1号车真实状态输出
    xo1 = x1 + 2*randn(3,1);               %1号车的观测状态
    yo1 = c*xo1;                           %1号车的观测器输出  
    r1=rand(1);r2=rand(1);  

    % 存储容器
    X1 = cell(1, 3000);    % 存储真实状态历史   
    XO1 = cell(1, 3000);   % 存储观测状态历史
    Eo1 = cell(1, 3000);   % 存储观测误差历史   
    
    % 初始状态赋值
    X1{1} = x1;        % 使用大括号{}访问元胞内容
    XO1{1} = xo1;
    Eo1{1} = x1 - xo1;
    cnt = 2;                                %计数器
    %%
    % 时间步长
    persistent  last_t;
    if isempty(last_t)
        last_t = t;
    end
    dt = t - last_t;                        %本次时间步长
    %%
    %{
       定义发生网络攻击的概率；
       分别为控制器受到的DoS攻击概率P1，观测器受到的DoS攻击概率P2、受到的FDI攻击P3;
       attack为攻击指示信号。
    %}
    p1 = 0.1; p2 = 0.1; p3 = 0.1;
    % 攻击指示信号
    attack1 = binornd(1, p1); attack2 = binornd(1, p2); attack3 = binornd(1, p3); 
    %%
    %{ 
        拉普拉斯矩阵+领导通信
       求解增益矩阵,定义状态权重矩阵 Q 和控制输入权重矩阵 R

    %}
    %
    Lg=[1+1 -1 0 0 0 0
        -1 2+1 -1 0 0 0 %
        0 -1 2+1 -1 0 0
        0 0 -1 2+1 -1 0
        0 0 0 -1 2+1 -1
        0 0 0 0  -1 1+1];
    % 求解增益矩阵
%     coder.extrinsic('setlmis')
%     coder.extrinsic('lmivar')
%     coder.extrinsic('lmiterm')
%     coder.extrinsic('getlmis')
%     coder.extrinsic('feasp')
%     coder.extrinsic('dec2mat')
%     setlmis([])
%     P1=lmivar(1,[3 1]);
%     H1=lmivar(2,[m 3]);
%     lmiterm([1 1 1 P1],A',1,'s');
%     lmiterm([1 1 1 H1],c',-1,'s');
%     lmiterm([2 1 1 P1],-1,1);
%     lmis=getlmis;
%     [tmin,xfeas]=feasp(lmis);
%     P=dec2mat(lmis,xfeas,P1);
%     P=P/1;  % 后续要用
%     L=dec2mat(lmis,xfeas,H1);
%     Lc=inv(P)*L';
%     SS=P*(A-Lc*c)+(A-Lc*c)'*P;
%     r=min(eig(Lg+Lg));
%     R=(1/r)*eye(size(B,2));
%     Q=0.5*eye(3);
%     M=care(A,B,Q,R);
%     K=-B'*M;    % 后续要用
%     S=2*eye(6); % 后续要用
%     D=kron(S,A)+kron(Lg,B*K);
%     D1=kron(S,M)*D+D'*kron(S,M);
      % 求解结果
      K = [-0.5,-1.3561,-0.6889];
      M = [1.3561,1.5889,0.5400;
            1.5889,3.7692,1.4645;
            0.5400,1.4645,0.7440];
      S=2*eye(6);
      P = diag([3.7797,3.7797,3.7797])*1.0e+08;
      Lc = [
            0.5000    0.5000   -0.0000;
            0.5000    0.5000    0.5000;
            0.0000    0.5000   -1.1667
             ];
    %%
    %{
        FRBNN参数设定以及函数设定
    %}
    num_memberships = 10;
    nums1 = 30 ; nums2 = 15;
    c1 = linspace(0, nums1, num_memberships);           % num_memberships中心值
    c2 = linspace(0, nums2, num_memberships); 
    c3 = [c1; c2];                                      % 两输入变量的中心
    bj = [3,1.5];
%   load('w.mat');
    w = [
        89.2059;
        81.0030;
        67.8877;
        48.4984;
        28.0749;
        2.5519;
        -18.6294;
        -51.9040;
        -65.3116;
        -136.9764;
        88.6140;
        81.6362;
        62.5570;
        40.9089;
        18.9510;
        -7.3399;
        -29.7779;
        -65.7111;
        -73.6754;
        -155.9809;
        79.3532;
        70.0337;
        51.2421;
        29.6544;
        7.2318;
        -17.3239;
        -40.1592;
        -72.2523;
        -81.0242;
        -155.6658;
        74.0738;
        63.1271;
        42.1875;
        20.5434;
        -1.8842;
        -25.8223;
        -47.6011;
        -79.0385;
        -85.0623;
        -165.9921;
        67.5292;
        56.4949;
        33.8765;
        12.7810;
        -9.2750;
        -33.3927;
        -52.4847;
        -85.3255;
        -85.1016;
        -171.6077;
        53.5968;
        49.2398;
        30.5450;
        6.0783;
        -17.3199;
        -41.3344;
        -65.9941;
        -86.1221;
        -110.7557;
        -163.5194;
        2.3790;
        2.3811;
        1.9368;
        1.1685;
        0.4642;
        -0.2833;
        -1.1271;
        -1.8114;
        -2.8696;
        -3.9755;
        1.0039;
        1.0041;
        1.0029;
        1.0005;
        0.9984;
        0.9961;
        0.9935;
        0.9914;
        0.9879;
        0.9850;
        1.0000;
        1.0000;
        1.0000;
        1.0000;
        1.0000;
        1.0000;
        1.0000;
        1.0000;
        1.0000;
        1.0000;
        1.0000;
        1.0000;
        1.0000;
        1.0000;
        1.0000;
        1.0000;
        1.0000;
        1.0000;
        1.0000;
        1.0000
    ];
    W=repmat(w,1,6);
    W=ones(num_memberships^2,6);
    W_1=W;W_2=zeros(num_memberships^2,6);
    beta1=flip(linspace(1e-5,1e-4,3000));
    beta=0.0005;
    alph=0.00005;
    % 神经网络函数模块
    function [ym,f3]=FRBNNout(x1,x2,c,bj,w_1,h)
        net2 = zeros(2,h);
        f2 = zeros(2,h);
        m1 = zeros(h);
        m2 = zeros(h);
        ff3 = zeros(h,h);
        % 输入层
        x=[x1,x2]';                    
        f1=x;
        % 模糊层
        for i=1:1:2                         
            for j=1:1:h
                net2(i,j)=-(f1(i)-c(i,j))^2/bj(i)^2;
            end
        end
        for i=1:1:2
            for j=1:1:h
                f2(i,j)=exp(net2(i,j));
            end
        end
        % 模糊推理层
        for j=1:1:h                       
            m1(j)=f2(1,j);
            m2(j)=f2(2,j);
        end
        
        for i=1:1:h
            for j=1:1:h
                ff3(i,j)=(m2(i)+m1(j))/2;
            end
        end
        % f3=[ff3(1,:),ff3(2,:),ff3(3,:),ff3(4,:),ff3(5,:)]';
        f3=reshape(ff3',[h^2,1]);
        % 输出层
        f4=w_1'*f3;                      
        ym=f4;
    end
    %%
    %{
        迭代；
        1 定义观测器受到的攻击
        2 定义观测器受攻击后的系统输出
        3 定义状态更新与控制更新 
        4 定义受到攻击的控制器
        5 
    %}
    % 传感器受到攻击后的输出
    
    if attack1 == 1
        y = zeros(3,1);     % 受到DoS攻击后值为0
        yo = zeros(3,1);    % 同上
    end
    % 非线性扰动项
    f = -(kd*(x1(2,1)^2)+kd*x1(2,1)*x1(3,1)-dm1)/m;   
    [fs,phi] = FRBNNout(xo1(2,1),xo1(3,1),c3,bj,W(:,1),num_memberships); % 神经网络 输入：v,a,c3,bj,w colum:i ,num
    S1 = r1*Bn*Bn'*P*(y1(1:3,1)-yo1(1:3,1))/norm(Bn'*P*(y1(1:3,1)-yo1(1:3,1))); %鲁棒项
    % 部分参数要修改 如x0
%     a1 = -r2*B'*M*(xo1(1:3,1)-car1_ref(1:3,1))/norm(B'*M*(xo1(1:3,1)-car1_ref(1:3,1))); % 估计误差的滑膜鲁棒项
    a1 =50; 
    a2 = 24;
%     a2 = -B'*M*(xo1(1:3,1)-car1_ref(1:3,1))*((xo1(1:3,1)-car1_ref(1:3,1))'*M*(Lc*c*(xo1(1:3,1)-x1(1:3,1))))/(norm(B'*M*(xo1(1:3,1)-car1_ref(1:3,1)))^2); 
    a=a1+a2;

    % 引入其它车辆的状态
    xo2 = [position2;v2;0];
    xo0 = [position0;v0;0];
    error_leader = 2*(xo0 - xo1);  % 与领导者的连接权重为2
    error_neighbor = -1*(xo2 - xo1);    % 与第二辆车的连接权重为-1
    % 控制器受到攻击后的输出
    if attack2 == 1
        u1 = K * (error_leader + error_neighbor); %分布式计算
    else
        u1 = 0;
    end
    if attack3 == 1
        u2 = sin(last_t);
    else 
        u2 = 0;
    end
    u = u1 + u2;  % 分组和并

    % 状态量更新
%     x1 = x1 + dt*(kron(S,A)*x1+kron(S,B)*u); %真实状态
%     xo1 = xo1 + dt*(kron(S,A)*xo1+kron(S,B)*u-kron(S,Lc)*(yo1-y1)); %观测状态
    x1 = x1 + dt*(2*A*xo0-A*xo2+2*B*u); 
%     car1_ref = car1_ref + dt*(kron(S,A)*car1_ref);
    car1_ref_dot = 2 * A .* car1_ref;  % 仅考虑与领导者的连接
    car1_ref = car1_ref + dt * car1_ref_dot;

    % 权重参数更新
    W(:,1)=W_1(:,1)+beta*f-fs*phi+alph*(W_1(:,1)-W_2(:,1));
    r1=r1+dt*((1/p1)*norm(Bn'*P*(y1(1:3,1)-yo1(1:3,1))));

    % 提取当前观测状态 (使用花括号{}访问元胞内容)
    current_xo1 = XO1{cnt-1};  % 假设cnt从2开始，cnt-1对应上一时间步
    
    % 计算r2更新
    r2 = r2 + dt * norm( B'*M*(x1(1:3,1) - current_xo1) );
%   r2=r2+dt*(norm(B'*M*(x1(1:3,1)-XO1(1:3,1))));

    W_1=W;
    W_2=W_1;
    
    % 实时输出端口
    position1 = x1(1); %位置输出
    v1 = x1(2);       %速度输出
    % 计数器+1
    cnt = cnt+1;
end

== matlab function paper1_cs/MATLAB Function ==
  data: position0 output; t input; v0 output; t output
function [position0,v0,t]= fnc(t)
    %虚拟领导者
    %计算时间步长
    position0 = 150;v0 = 20;a0 = 0;
    persistent last_t;
    if isempty(last_t)
        last_t = t;  % 初始化时间
    end
    dt = t - last_t;  % 计算时间步长
    position0 = position0 + v0*dt;
  
%     % 初始化持久变量
%     persistent p_lst v_lst last_t init_flag
%     if isempty(init_flag)  % 首个仿真步
%         p_lst = 150; 
%         v_lst = 20; 
%         last_t = t;
%         init_flag = true;
%     end
%     
%     dt = t - last_t;       % 时间步长计算
%     if dt < eps            % 预防仿真器时间重叠
%         dt = 0.01;         % 预定义名义步长替代 (根据实际设定)
%     end
% 
%     p0 = p_lst + v_lst*dt + 0.5*0*dt^2; %动力学积分(假设无加速度)
%     v0 = v_lst;  
%     p_lst = p0;            %更新位姿状态
%     last_t = t;            %记录本次时刻
end

== matlab function paper1_cs/分布式控制器 ==
  data: p1 output; p2 output; p3 output; p4 output; p5 output; p6 output; time input; v1 output; v2 output; v3 output; v4 output; v5 output; v6 output; as1 output; as2 output; as3 output; as4 output; as5 output; as6 output; ep1 output; ep2 output; ep3 output; ep4 output; ep5 output; ep6 output; ev1 output; ev2 output; ev3 output; ev4 output; ev5 output; ev6 output; ea1 output; ea2 output; ea3 output; ea4 output; ea5 output; ea6 output; lep1 output; lep2 output; lep3 output; lep4 output; lep5 output; lep6 output; lev1 output; lev2 output; lev3 output; lev4 output; lev5 output; lev6 output; lea1 output; lea2 output; lea3 output; lea4 output; lea5 output; lea6 output
function [p1,p2,p3,p4,p5,p6,v1,v2,v3,v4,v5,v6,as1,as2,as3,as4,as5,as6,ep1,ep2,ep3,ep4,ep5,ep6,ev1,ev2,ev3,ev4,ev5,ev6,ea1,ea2,ea3,ea4,ea5,ea6,lep1,lep2,lep3,lep4,lep5,lep6...
    ,lev1,lev2,lev3,lev4,lev5,lev6,lea1,lea2,lea3,lea4,lea5,lea6] = fcn(time)    
    
    % 定义持久变量
    persistent x xo u W r1 r2 f fs phi AS Bs y yo a1 a2 X0 X1 x0 S1
    
    m=1.8;%质量
    Tau=0.6;%时滞常数
    le=5;%车辆长度
    A=[0 1 0; 0 0 1; 0 0 -1/Tau];%系统状态矩阵
    ds=15;%期望距离
    B=[0;0;1/(m*Tau)];%控制输入矩阵
    Bn=[0;0;1];
    B1=kron(eye(6),Bn);
    kd1=0.24;kd2=0.25;kd3=0.23;kd4=0.21;kd5=0.22;kd6=0.22;
    kd=[kd1;kd2;kd3;kd4;kd5;kd6];
    dm1=124.9;dm2=116.4;dm3=125.4;dm4=117.7;dm5=120.5;dm6=121.5;
    dm=[dm1;dm2;dm3;dm4;dm5;dm6];
    % c=rand(2,3);
    c=eye(3);
    % c=[1 0 1;0 1 0];
    C=kron(eye(6),c); % expand
    m=size(c,1);    
    %%
    t=0.01;%步长
    T=120;%总仿真时长
    k=size((0:t:T),2)-1;%仿真迭代次数
    % 预先分配
    Ti = zeros(1,k);
    X1 = zeros(18,1);
    % 初始状态值
    p0=150;v0=20;a0=0;

    if isempty(x0)
        x0=[p0;v0;a0];%leader
    end
%     x0 = x0 + [v0; a0; 0] * t;

%     if isempty(X1)
        for j=1:3:18
            X1(j:j+2,1)=[le+(1+(j-1)/3)*ds;0;0]; % 用于计算每辆车相对于 leader 的期望状态
        end
%     end
    
    %领导车
    if isempty(X0)
        X0=repmat(x0,6,1)-X1;
    end

    if isempty(x)
        x = [120; 10; 2; 100; 4; 3; 80; 7; 3; 60; 11; 1; 40; 9; 0.5; 20; 3; 0.6];
        y=C*x;
        xo=x+2*randn(18,1);%观测器状态
        yo=C*xo;
    end
    
    
    %定义元胞数组、存储数据
    X=cell(1,k);Xo=cell(1,k);Eo=cell(1,k);Ec=cell(1,k);
    X{1,1}={x};Xo{1,1}={xo};Eo{1,1}={x-xo};
    Ec{1,1}={x-X0};
    r1=rand(6,1);r2=rand(6,1);
    F=cell(1,k);Fs=cell(1,k);
    %%
    %随机攻击信号设置
    %攻击期望状态
    % 伯努利分布函数
    function bernoulli_samples = gBernoulli(num_samples, p)
        if p < 0 || p > 1
            error('p illega');
        end
        % 生成伯努利分布样本
        bernoulli_samples = rand(num_samples, 1) < p;
    end    

    alpoe1=0.9999;alpoe2=1;alpoe3=0.99996;alpoe4=0.99998;alpoe5=0.99999;alpoe6=0.99996;
    Dos1=[alpoe1,alpoe2,alpoe3,alpoe4,alpoe5,alpoe6];
    %攻击状态随机生成
    alpo1=gBernoulli(k,alpoe1);alpo2=gBernoulli(k,alpoe2);alpo3=gBernoulli(k,alpoe3);alpo4=gBernoulli(k,alpoe4);alpo5=gBernoulli(k,alpoe5);alpo6=gBernoulli(k,alpoe6);
    %控制器DOS攻击
    alpce1=0.95;alpce2=0.9999;alpce3=0.95;alpce4=0.95;alpce5=0.95;alpce6=0.95;
    Dos2=[alpce1,alpce2,alpce3,alpce4,alpce5,alpce6];
    %控制器DOS攻击随机数生成
    alpc1=gBernoulli(k,alpce1);alpc2=gBernoulli(k,alpce2);alpc3=gBernoulli(k,alpce3);alpc4=gBernoulli(k,alpce4);alpc5=gBernoulli(k,alpce5);alpc6=gBernoulli(k,alpce6);
    %FDI攻击期望
    betce1=0.5;betce2=0.5;betce3=0.5;betce4=0.5;betce5=0.5;betce6=0.5;
    FDI=[betce1,betce2,betce3,betce4,betce5,betce6];
    %DFI攻击随机数生成
    betc1=gBernoulli(k,betce1);betc2=gBernoulli(k,betce2);betc3=gBernoulli(k,betce3);betc4=gBernoulli(k,betce4);betc5=gBernoulli(k,betce5);betc6=gBernoulli(k,betce6);
    %%
    %拉普拉斯矩阵+领导通信
    Lg=[1+1 -1 0 0 0 0
        -1 2+1 -1 0 0 0 %
        0 -1 2+1 -1 0 0
        0 0 -1 2+1 -1 0
        0 0 0 -1 2+1 -1
        0 0 0 0  -1 1+1];
      K = [-0.5,-1.3561,-0.6889];
      M = [1.3561,1.5889,0.5400;
            1.5889,3.7692,1.4645;
            0.5400,1.4645,0.7440];
      S=2*eye(6);
      P = diag([3.7797,3.7797,3.7797])*1.0e+08;
      Lc = [
            0.5000    0.5000   -0.0000;
            0.5000    0.5000    0.5000;
            0.0000    0.5000   -1.1667
             ];
    %%
    %FRBNN函数
    function [ym,f3]=FRBNNout(x1,x2,c,bj,w_1,h)
        net2 = zeros(2,h);
        f2 = zeros(2,h);
        m1 = zeros(h);
        m2 = zeros(h);
        ff3 = zeros(h,h);
        xn=[x1,x2]';                     % Layer1:input
        
        f1=xn;
        %%%%%%%%%%%%%%%%%%%%%%%%%%%%%%%%%%%%%%%%%%%%%%%%%%%%%%%
        for i=1:1:2                         % Layer2:fuzzation
            for j=1:1:h
                net2(i,j)=-(f1(i)-c(i,j))^2/bj(i)^2;
            end
        end
        for i=1:1:2
            for j=1:1:h
                f2(i,j)=exp(net2(i,j));
            end
        end
        %%%%%%%%%%%%%%%%%%%%%%%%%%%%%%%%%%%%%%%%%%%%%%%%%%%%%%%
        for j=1:1:h                       % Layer3:fuzzy inference(25 rules)
            m1(j)=f2(1,j);
            m2(j)=f2(2,j);
        end
        
        for i=1:1:h
            for j=1:1:h
                ff3(i,j)=(m2(i)+m1(j))/2;
            end
        end
        % f3=[ff3(1,:),ff3(2,:),ff3(3,:),ff3(4,:),ff3(5,:)]';
        f3=reshape(ff3',[h^2,1]);
        %%%%%%%%%%%%%%%%%%%%%%%%%%%%%%%%%%%%%%%%%%%%%%%%%%%%%%%
        
        f4=w_1'*f3;                      % Layer4:output
        ym=f4;
    end

    %FRBFNN参数
    num_memberships = 10;
    nums1 = 30 ; nums2 = 15;
    c1 = linspace(0, nums1, num_memberships); % num_memberships中心值
    c2 = linspace(0, nums2, num_memberships); 
    c3 = [c1; c2]; % 两输入变量的中心
    bj = [3,1.5];
%     W=repmat(w,1,6);
    W=ones(num_memberships^2,6);
    persistent W_1 W_2
    if isempty(W_1)
        W_1=W;
    end
    if isempty(W_2)
        W_2=zeros(num_memberships^2,6);
    end
    beta1=flip(linspace(1e-5,1e-4,k));
    beta=0.0005;
    alph=0.00005;
    %%
    %迭代
    %需要初始化的变量 
    if isempty(f)
        f = zeros(6,1);fs = zeros(6,1);phi = zeros(100,6);S1 = zeros(18,6); a1 = zeros(6,1);a2 = zeros(6,2);
    end

    persistent gi
    if isempty(gi)
        gi = 0; % 初始化 i
    end
    gi = gi + 1;  % i 递增
    
    Os=diag([alpo1(gi),alpo2(gi),alpo3(gi),alpo4(gi),alpo5(gi),alpo6(gi)],0);%输出DoS攻击信号

    y=kron(Os,eye(3))*(C*x);                %受到攻击后实际系统输出
    yo=kron(diag(Dos1,0),eye(3))*(C*xo);
    
    % size(k)
    for j=1:3:18
        
    f(1+(j-1)/3,1)=-(kd(1+(j-1)/3)*(x(j+1,1)^2)+kd(1+(j-1)/3)*x(j+1,1)*x(j+2,1)-dm(1+(j-1)/3))/m; %非线性扰动
        
        [fs(1+(j-1)/3,1),phi(:,1+(j-1)/3)]=FRBNNout(xo(j+1,1),xo(j+2,1),c3,bj,W(:,1+(j-1)/3),num_memberships); % 神经网络输出与径向基函数输出
        FRBNNout(xo(j+1,1),xo(j+2,1),c3,bj,W(:,1+(j-1)/3),num_memberships);
        S1(j:j+2,1)=r1(1+(j-1)/3,1)*Bn*Bn'*P*(y(j:j+2,1)-yo(j:j+2,1))/norm(Bn'*P*(y(j:j+2,1)-yo(j:j+2,1))); % 鲁棒项

        a1(1+(j-1)/3,1)=-r2(1+(j-1)/3,1)*B'*M*(xo(j:j+2,1)-X0(j:j+2,1))/norm(B'*M*(xo(j:j+2,1)-X0(j:j+2,1))); % 估计误差的滑膜鲁棒项
        a2(1+(j-1)/3,1)=-B'*M*(xo(j:j+2,1)-X0(j:j+2,1))*((xo(j:j+2,1)-X0(j:j+2,1))'*M*(Lc*c*(xo(j:j+2,1)-x(j:j+2,1))))/(norm(B'*M*(xo(j:j+2,1)-X0(j:j+2,1)))^2);
        a=a1+a2;
    end

    % u=(kron(Lg,K)*(xo-X0)+a);
    % 控制器受到的攻击
    AS=diag([alpc1(gi),alpc2(gi),alpc3(gi),alpc4(gi),alpc5(gi),alpc6(gi)],0); %控制器DoS攻击信号 
    Bs=[betc1(gi);betc2(gi);betc3(gi);betc4(gi);betc5(gi);betc6(gi)];         %控制器FDI攻击信号
    % u=AS*(kron(Lg,K)*(xo-X0)+a)+Bs*sin(t*i);
    AS*kron(Lg,K)*(xo-X0);

    u=AS*(kron(Lg,K)*(xo-X0))+Bs*sin(time);
    
    if time<=60
       X0=X0+t*(kron(S,A)*X0);
%        (kron(S,A)*X0)
    end
    if time>60 && time<=90
       X0=X0+t*(kron(S,A)*X0+repmat([0;1;0],6,1));
%        (kron(S,A)*X0+repmat([0;1;0],6,1))
    end
    if time>90
       X0=X0+t*(kron(S,A)*X0);
%        (kron(S,A)*X0)
    end


    %%
    % 对比试验u
    %%
    % +kron(S,B)*u   +kron(eye(6),Bn)*f

    % x=x+t*(kron(S,A)*x+kron(S,B)*u+kron(eye(6),Bn)*f);
    % xo=xo+t*(kron(S,A)*xo+kron(S,B)*u-kron(S,Lc)*(yo-y)+kron(eye(6),Bn)*fs);
    x=x+t*(kron(S,A)*x+kron(S,B)*u);
    xo=xo+t*(kron(S,A)*xo+kron(S,B)*u-kron(S,Lc)*(yo-y));
    


    for j=1:3:18
        % W(:,1+(j-1)/3)=W(:,1+(j-1)/3)+t*(Bn'*P*(y(j:j+2,1)-yo(j:j+2,1)));

      W(:,1+(j-1)/3)=W_1(:,1+(j-1)/3)+beta*(f(1+(j-1)/3,1)-fs(1+(j-1)/3,1))*phi(:,1+(j-1)/3)+alph*(W_1(:,1+(j-1)/3)-W_2(:,1+(j-1)/3));


        r1(1+(j-1)/3,1)=r1(1+(j-1)/3,1)+t*((1/Dos1(1+(j-1)/3))*norm(Bn'*P*(y(j:j+2,1)-yo(j:j+2,1))));
        % r2(1+(j-1)/3,1)=r2(1+(j-1)/3,1)+t*(norm(B'*M1*(xo(j:j+2,1)-X0(j:j+2,1))));
        r2(1+(j-1)/3,1)=r2(1+(j-1)/3,1)+t*(norm(B'*M*(x(j:j+2,1)-X0(j:j+2,1))));
    end

    
%     X(1,i+1)={x};
%     Xo(1,i+1)={xo};
% 
%     Eo(1,i+1)= {x-xo};
%     Ec(1,i+1)={x-X0}; 
%     Ti(i+1)=t*i;
%     F(1,i)={f};
%     Fs(1,i)={fs};
    %输出数据     
    p1 = x(1,1);
    v1 = x(2,1);
    as1 = x(3,1);

    p2 = x(4, 1);
    v2 = x(5, 1);
    as2 = x(6, 1);

    p3 = x(7, 1);
    v3 = x(8, 1);
    as3 = x(9, 1);
    
    p4 = x(10, 1);
    v4 = x(11, 1);
    as4 = x(12, 1);
    
    p5 = x(13, 1);
    v5 = x(14, 1);
    as5 = x(15, 1);
    
    p6 = x(16, 1);
    v6 = x(17, 1);
    as6 = x(18, 1);

    p1o = xo(1, 1);  % 提取 xo 的第一个元素
    v1o = xo(2, 1);  % 提取 xo 的第二个元素
    as1o = xo(3, 1); % 提取 xo 的第三个元素
    
    p2o = xo(4, 1);  % 提取 xo 的第四个元素
    v2o = xo(5, 1);  % 提取 xo 的第五个元素
    as2o = xo(6, 1); % 提取 xo 的第六个元素
    
    p3o = xo(7, 1);  % 提取 xo 的第七个元素
    v3o = xo(8, 1);  % 提取 xo 的第八个元素
    as3o = xo(9, 1); % 提取 xo 的第九个元素
    
    p4o = xo(10, 1); % 提取 xo 的第十个元素
    v4o = xo(11, 1); % 提取 xo 的第十一个元素
    as4o = xo(12, 1); % 提取 xo 的第十二个元素
    
    p5o = xo(13, 1); % 提取 xo 的第十三个元素
    v5o = xo(14, 1); % 提取 xo 的第十四个元素
    as5o = xo(15, 1); % 提取 xo 的第十五个元素
    
    p6o = xo(16, 1); % 提取 xo 的第十六个元素
    v6o = xo(17, 1); % 提取 xo 的第十七个元素
    as6o = xo(18, 1); % 提取 xo 的第十八个元素
    

    %   观测器与真实状态的误差曲线
    % 定义误差变量
    ep1 = p1 - p1o; % 车辆 1 与虚拟领导者的位置误差
    ev1 = v1 - v1o; 
    ea1 = as1 - as1o; 
    
    ep2 = p2 - p2o; 
    ev2 = v2 - v2o; 
    ea2 = as2 - as2o; 
    
    ep3 = p3 - p3o; 
    ev3 = v3 - v3o; 
    ea3 = as3 - as3o; 
    
    ep4 = p4 - p4o;
    ev4 = v4 - v4o; 
    ea4 = as4 - as4o; 
    
    ep5 = p5 - p5o;
    ev5 = v5 - v5o;
    ea5 = as5 - as5o; 
    
    ep6 = p6 - p6o; 
    ev6 = v6 - v6o; 
    ea6 = as6 - as6o; 
       
    %%
    % 领导者与跟随车之间的误差
    % 位置
    lep1 = X0(1,1) - p1; % 车辆 1 与虚拟领导者的期望位置误差
    lep2 = X0(4,1) - p2; % 车辆 2 与虚拟领导者的期望位置误差
    lep3 = X0(7,1) - p3; % 车辆 3 与虚拟领导者的期望位置误差
    lep4 = X0(10,1) - p4; % 车辆 4 与虚拟领导者的期望位置误差
    lep5 = X0(13,1) - p5; % 车辆 5 与虚拟领导者的期望位置误差
    lep6 = X0(16,1) - p6; % 车辆 6 与虚拟领导者的期望位置误差

    lev1 = v1o - v1; % 车辆 1 与虚拟领导者的速度误差
    lev2 = v2o - v2; % 车辆 2 与虚拟领导者的速度误差
    lev3 = v3o - v3; % 车辆 3 与虚拟领导者的速度误差
    lev4 = v4o - v4; % 车辆 4 与虚拟领导者的速度误差
    lev5 = v5o - v5; % 车辆 5 与虚拟领导者的速度误差
    lev6 = v6o - v6; % 车辆 6 与虚拟领导者的速度误差

    lea1 = as1o - as1; % 车辆 1 与虚拟领导者的加速度误差
    lea2 = as2o - as2; % 车辆 2 与虚拟领导者的加速度误差
    lea3 = as3o - as3; % 车辆 3 与虚拟领导者的加速度误差
    lea4 = as4o - as4; % 车辆 4 与虚拟领导者的加速度误差
    lea5 = as5o - as5; % 车辆 5 与虚拟领导者的加速度误差
    lea6 = as6o - as6; % 车辆 6 与虚拟领导者的加速度误差
end
